simulink library "mag_PD_control_new"  (R2016b)
settings: Solver=VariableStepAuto  StartTime=0.0  StopTime=10.0  RelTol=1e-3
undefined symbols (not defined in the file or in its folder): fsw_params
libraries: vrlib x2, aerolibutil x2
settings Model: Creator=taylorreynolds  LastModifiedBy=evich

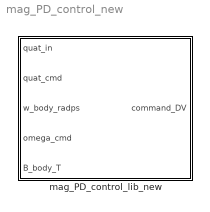
== system mag_PD_control_new ==
  "mag_PD_control_lib_new " : Subsystem

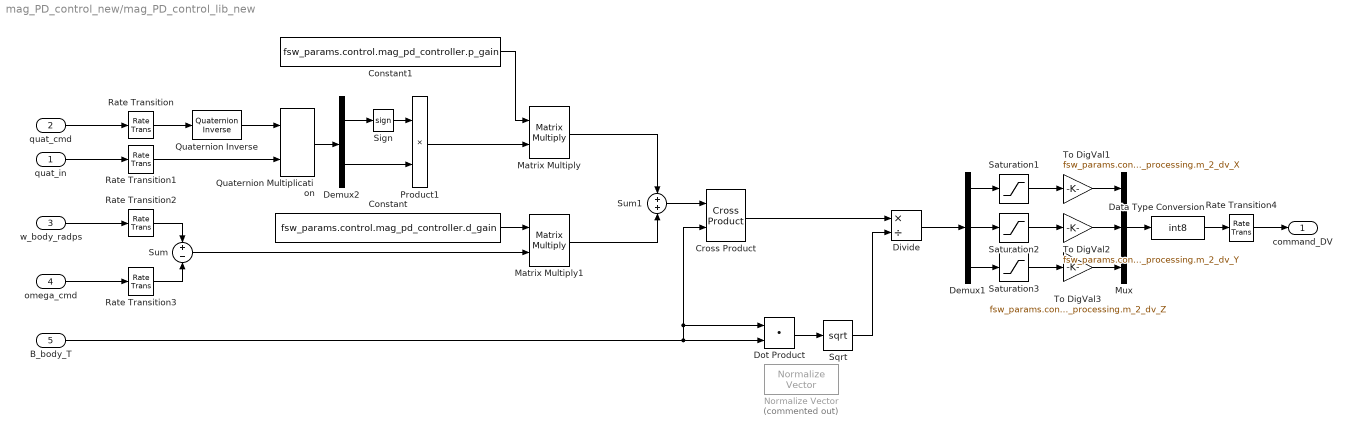
== system mag_PD_control_new/mag_PD_control_lib_new  ==
  quat_in : Inport
  quat_cmd : Inport  Port=2
  w_body_radps : Inport  Port=3
  omega_cmd : Inport  Port=4
  B_body_T : Inport  Port=5
  Constant : Constant  Value=fsw_params.control.mag_pd_controller.d_gain
  Constant1 : Constant  Value=fsw_params.control.mag_pd_controller.p_gain
  Cross Product : vrlib/Utilities/Cross Product
  Data Type Conversion : DataTypeConversion  OutDataTypeStr=int8
  Demux1 : Demux  Outputs=3
  Demux2 : Demux  Outputs=[1 3]
  Divide : Product  Inputs=*/
  Dot Product : DotProduct  InputSameDT=on  OutDataTypeStr=Inherit: Inherit via internal rule
  Matrix Multiply : Product  Multiplication=Matrix(*)
  Matrix Multiply1 : Product  Multiplication=Matrix(*)
  Mux : Mux  Inputs=3
  Normalize Vector : vrlib/Utilities/Normalize Vector  Commented=on  maxzero=0
  Product1 : Product
  Quaternion Inverse : aerolibutil/Quaternion Inverse
  Quaternion Multiplication : aerolibutil/Quaternion Multiplication
  Rate Transition{,1..3} (4 alike) : RateTransition  OutPortSampleTime=fsw_params.control.mag_pd_controller.sample_time_s
  Rate Transition4 : RateTransition
  Saturation1 : Saturate  UpperLimit=fsw_params.actuators.magnetorquer.max_dipole_x  LowerLimit=-fsw_params.actuators.magnetorquer.max_dipole_x
  Saturation2 : Saturate  UpperLimit=fsw_params.actuators.magnetorquer.max_dipole_y  LowerLimit=-fsw_params.actuators.magnetorquer.max_dipole_y
  Saturation3 : Saturate  UpperLimit=fsw_params.actuators.magnetorquer.max_dipole_z  LowerLimit=-fsw_params.actuators.magnetorquer.max_dipole_z
  Sign : Signum
  Sqrt : Sqrt  SaturateOnIntegerOverflow=on
  Sum : Sum  Inputs=+-
  Sum1 : Sum
  To DigVal1 : Gain  Gain=fsw_params.control.cmd_processing.m_2_dv_X
  To DigVal2 : Gain  Gain=fsw_params.control.cmd_processing.m_2_dv_Y
  To DigVal3 : Gain  Gain=fsw_params.control.cmd_processing.m_2_dv_Z
  command_DV : Outport
  wires:
  quat_in/1 -> Rate Transition1/1
  w_body_radps/1 -> Rate Transition2/1
  omega_cmd/1 -> Rate Transition3/1
  quat_cmd/1 -> Rate Transition/1
  Rate Transition4/1 -> command_DV/1
  Demux1/1 -> Saturation1/1
  Demux1/3 -> Saturation3/1
  Demux1/2 -> Saturation2/1
  Saturation1/1 -> To DigVal1/1
  Saturation2/1 -> To DigVal2/1
  Saturation3/1 -> To DigVal3/1
  Mux/1 -> Data Type Conversion/1
  To DigVal3/1 -> Mux/3
  To DigVal2/1 -> Mux/2
  To DigVal1/1 -> Mux/1
  Data Type Conversion/1 -> Rate Transition4/1
  B_body_T/1 -> Cross Product/2, Dot Product/1, Dot Product/2
  Rate Transition2/1 -> Sum/1
  Rate Transition3/1 -> Sum/2
  Rate Transition1/1 -> Quaternion Multiplication/2
  Rate Transition/1 -> Quaternion Inverse/1
  Quaternion Inverse/1 -> Quaternion Multiplication/1
  Matrix Multiply1/1 -> Sum1/2
  Quaternion Multiplication/1 -> Demux2/1
  Matrix Multiply/1 -> Sum1/1
  Sign/1 -> Product1/1
  Demux2/1 -> Sign/1
  Constant/1 -> Matrix Multiply1/1
  Constant1/1 -> Matrix Multiply/1
  Demux2/2 -> Product1/2
  Sum/1 -> Matrix Multiply1/2
  Dot Product/1 -> Sqrt/1
  Sqrt/1 -> Divide/2
  Cross Product/1 -> Divide/1
  Product1/1 -> Matrix Multiply/2
  Sum1/1 -> Cross Product/1
  Divide/1 -> Demux1/1
